simulink model "CHB_3phaseSVPWM_Phaseshift"  (R2015a)
settings: Solver=ode45  StartTime=0.0  StopTime=0.2  MaxStep=0.000001  MinStep=0.0000001  RelTol=1e-3
libraries: powerlib x33, simulink x1
settings Model: Creator=hp  LastModifiedBy=hp

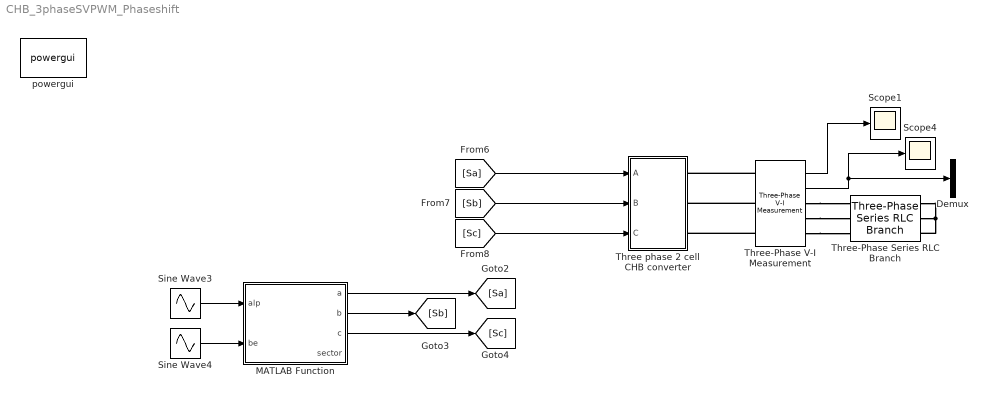
== system CHB_3phaseSVPWM_Phaseshift ==
  Demux : Demux  Outputs=3
  MATLAB Function : MATLAB Function  TreatAsAtomicUnit=on
  Scope1 : Scope
      settings: YMin=-400  YMax=400
  Scope4 : Scope
      settings: YMin=-22.5  YMax=22.5  SaveName=ScopeData5
  Sine Wave3 : Sin  Amplitude=1.0  Frequency=2*pi*50  SampleTime=0
  Sine Wave4 : Sin  Amplitude=1.0  Frequency=2*pi*50  Phase=pi/2  SampleTime=0
  Three phase 2 cell CHB converter : Subsystem
  Three-Phase Series RLC Branch : powerlib/Elements/Three-Phase Series RLC Branch  LConnTagsString=A|B|C  RConnTagsString=A|B|C  BranchType=RLC  Resistance=10  Inductance=10e-3  Capacitance=0  Measurements=None
  Three-Phase V-I Measurement : powerlib/Measurements/Three-Phase V-I Measurement  VoltageMeasurement=phase-to-phase  SetLabelV=off  LabelV=Vabc  Vpu=off  VpuLL=off  CurrentMeasurement=yes  SetLabelI=off  LabelI=Iabc  Ipu=off  Pbase=100e6  Vbase=500e3  OutputType=Complex  PhasorSimulation=off  PSBequivalent=0
  powergui : powerlib/powergui  Priority=1  SimulationMode=Continuous  SolverType=Tustin/Backward Euler (TBE)  SampleTime=50e-6  frequency=60  SPID=off  DisableSnubberDevices=off  DisableRonSwitches=off  DisableVfSwitches=off  SwTol=0  DisplayEquations=off  Interpol=off  methode=off  Ts=100  FunctionMessages=off  echomessages=off  HookPort=off  EnableUseOfTLC=off  x0status=blocks  frequencyindice=0  Pbase=100e6  ErrMax=1e-4  Iterations=50  UnitsV=kV  UnitsW=MW  buscounter=0  RestoreLinks=warning  ResistiveCurrentMeasurement=off  Frange=[0:2:500]  Ylog=off  Xlog=on  ShowGrid=off  save=off  variable=ZData  structure=0  ZoomFFT=off  StartTime=0.0  cycles=1  DisplayStyle=1  fundamental=60  FreqAxis=off  MaxFrequency=1000  frequencyindicesteady=1  RmsSteady=1  display=off
  wires:
  MATLAB Function/1(a) -> [Sa]
  MATLAB Function/2(b) -> [Sb]
  Sine Wave3/1 -> MATLAB Function/1(alp)
  Sine Wave4/1 -> MATLAB Function/2(be)
  MATLAB Function/3(c) -> [Sc]
  Three-Phase V-I Measurement/2 -> Scope4/1, Demux/1
  [Sa] -> Three phase 2 cell CHB converter/1(A)
  [Sb] -> Three phase 2 cell CHB converter/2(B)
  [Sc] -> Three phase 2 cell CHB converter/3(C)
  Three-Phase V-I Measurement/1 -> Scope1/1
  connections:
  Three-Phase Series RLC Branch/RConn1 -- Three-Phase Series RLC Branch/RConn2 -- Three-Phase Series RLC Branch/RConn3
  Three-Phase V-I Measurement/RConn1 -- Three-Phase Series RLC Branch/LConn1
  Three-Phase V-I Measurement/RConn2 -- Three-Phase Series RLC Branch/LConn2
  Three-Phase V-I Measurement/RConn3 -- Three-Phase Series RLC Branch/LConn3
  Three-Phase V-I Measurement/LConn1 -- Three phase 2 cell CHB converter/RConn1
  Three-Phase V-I Measurement/LConn2 -- Three phase 2 cell CHB converter/RConn2
  Three-Phase V-I Measurement/LConn3 -- Three phase 2 cell CHB converter/RConn3

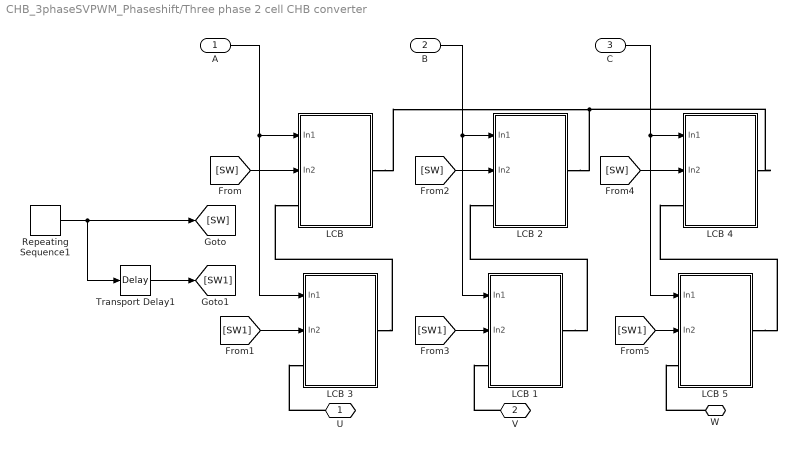
== system CHB_3phaseSVPWM_Phaseshift/Three phase 2 cell CHB converter ==
  A : Inport
  B : Inport  Port=2
  C : Inport  Port=3
  "LCB " : Subsystem
  LCB 1 : Subsystem
  LCB 2 : Subsystem
  LCB 3 : Subsystem
  LCB 4 : Subsystem
  LCB 5 : Subsystem
  Repeating Sequence1 : simulink/Sources/Repeating Sequence  rep_seq_t=[0 0.5 1]/1000  rep_seq_y=[0 1 0]
  Transport Delay1 : TransportDelay  DelayTime=1/4000
  U : PMIOPort  Port=1  Side=Right
  V : PMIOPort  Port=2  Side=Right
  W : PMIOPort  Port=3  Side=Right
  wires:
  [SW1] -> LCB 3/2(In2)
  [SW1] -> LCB 5/2(In2)
  A/1 -> LCB 3/1(In1), "LCB "/1(In1)
  [SW] -> LCB 2/2(In2)
  Repeating Sequence1/1 -> Transport Delay1/1, [SW]
  C/1 -> LCB 4/1(In1), LCB 5/1(In1)
  [SW] -> "LCB "/2(In2)
  [SW1] -> LCB 1/2(In2)
  Transport Delay1/1 -> [SW1]
  B/1 -> LCB 1/1(In1), LCB 2/1(In1)
  [SW] -> LCB 4/2(In2)
  connections:
  "LCB "/RConn1 -- LCB 4/RConn1 -- LCB 2/RConn1
  LCB 3/RConn1 -- "LCB "/LConn1
  LCB 1/RConn1 -- LCB 2/LConn1
  U/RConn1 -- LCB 3/LConn1
  LCB 5/RConn1 -- LCB 4/LConn1
  V/RConn1 -- LCB 1/LConn1
  W/RConn1 -- LCB 5/LConn1

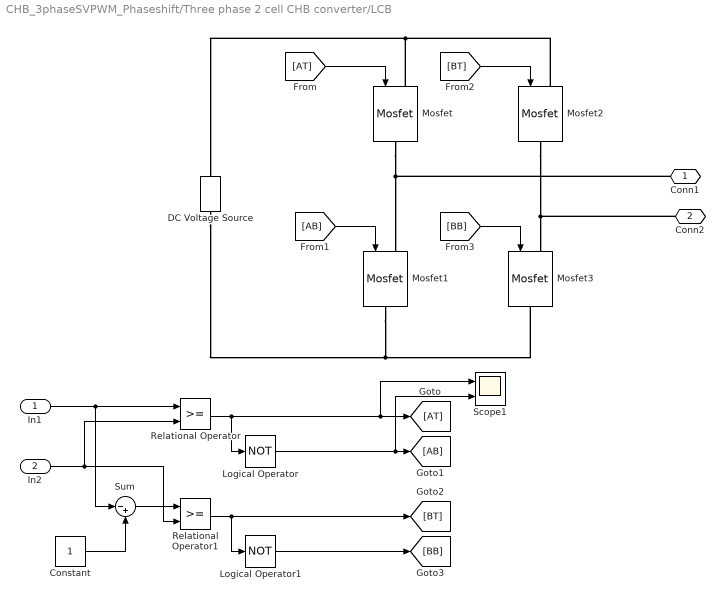
== system CHB_3phaseSVPWM_Phaseshift/Three phase 2 cell CHB converter/LCB  ==
  In1 : Inport
  In2 : Inport  Port=2
  Constant : Constant
  DC Voltage Source : powerlib/Electrical Sources/DC Voltage Source  Amplitude=100  Measurements=None
  Logical Operator : Logic  Operator=NOT  Inputs=1  AllPortsSameDT=off  OutDataTypeStr=boolean
  Logical Operator1 : Logic  Operator=NOT  Inputs=1  AllPortsSameDT=off  OutDataTypeStr=boolean
  Mosfet{,1..3} (4 alike) : powerlib/Power Electronics/Mosfet  Ron=0.1  Lon=0  Rd=0.01  Vfd=0  IC=0  Rs=1e5  Cs=inf  Measurements=off
  Relational Operator : RelationalOperator  OutDataTypeStr=boolean
  Relational Operator1 : RelationalOperator  OutDataTypeStr=boolean
  Scope1 : Scope  NumInputPorts=2
      settings: YMin=-80~-5  YMax=80~5
  Sum : Sum  Inputs=|-+
  Conn1 : PMIOPort  Port=1  Side=Right
  Conn2 : PMIOPort  Port=2  Side=Left
  wires:
  Sum/1 -> Relational Operator1/1
  Relational Operator/1 -> Scope1/1, [AT], Logical Operator/1
  Logical Operator/1 -> Scope1/2, [AB]
  Relational Operator1/1 -> [BT], Logical Operator1/1
  Logical Operator1/1 -> [BB]
  [BB] -> Mosfet3/1
  [AB] -> Mosfet1/1
  [AT] -> Mosfet/1
  [BT] -> Mosfet2/1
  In2/1 -> Relational Operator1/2, Relational Operator/2
  In1/1 -> Sum/1, Relational Operator/1
  Constant/1 -> Sum/2
  connections:
  Mosfet2/RConn1 -- Conn2/RConn1 -- Mosfet3/LConn1
  DC Voltage Source/LConn1 -- Mosfet1/RConn1 -- Mosfet3/RConn1
  Mosfet2/LConn1 -- Mosfet/LConn1 -- DC Voltage Source/RConn1
  Mosfet/RConn1 -- Conn1/RConn1 -- Mosfet1/LConn1

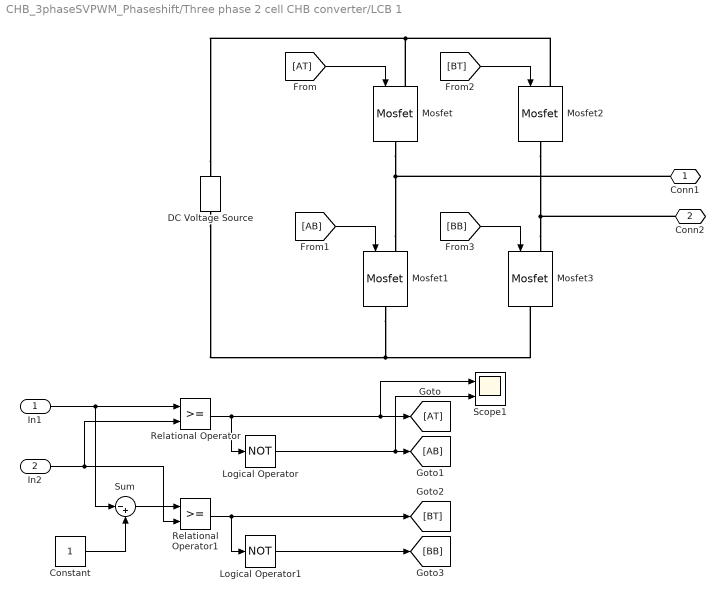
== system CHB_3phaseSVPWM_Phaseshift/Three phase 2 cell CHB converter/LCB 1 ==
  In1 : Inport
  In2 : Inport  Port=2
  Constant : Constant
  DC Voltage Source : powerlib/Electrical Sources/DC Voltage Source  Amplitude=100  Measurements=None
  Logical Operator : Logic  Operator=NOT  Inputs=1  AllPortsSameDT=off  OutDataTypeStr=boolean
  Logical Operator1 : Logic  Operator=NOT  Inputs=1  AllPortsSameDT=off  OutDataTypeStr=boolean
  Mosfet{,1..3} (4 alike) : powerlib/Power Electronics/Mosfet  Ron=0.1  Lon=0  Rd=0.01  Vfd=0  IC=0  Rs=1e5  Cs=inf  Measurements=off
  Relational Operator : RelationalOperator  OutDataTypeStr=boolean
  Relational Operator1 : RelationalOperator  OutDataTypeStr=boolean
  Scope1 : Scope  NumInputPorts=2
      settings: YMin=-80~-5  YMax=80~5
  Sum : Sum  Inputs=|-+
  Conn1 : PMIOPort  Port=1  Side=Right
  Conn2 : PMIOPort  Port=2  Side=Left
  wires:
  Constant/1 -> Sum/2
  In1/1 -> Relational Operator/1, Sum/1
  In2/1 -> Relational Operator/2, Relational Operator1/2
  [BT] -> Mosfet2/1
  [AT] -> Mosfet/1
  [AB] -> Mosfet1/1
  [BB] -> Mosfet3/1
  Logical Operator1/1 -> [BB]
  Relational Operator1/1 -> Logical Operator1/1, [BT]
  Logical Operator/1 -> [AB], Scope1/2
  Relational Operator/1 -> Logical Operator/1, [AT], Scope1/1
  Sum/1 -> Relational Operator1/1
  connections:
  Mosfet1/LConn1 -- Conn1/RConn1 -- Mosfet/RConn1
  DC Voltage Source/RConn1 -- Mosfet/LConn1 -- Mosfet2/LConn1
  Mosfet3/RConn1 -- Mosfet1/RConn1 -- DC Voltage Source/LConn1
  Mosfet3/LConn1 -- Conn2/RConn1 -- Mosfet2/RConn1

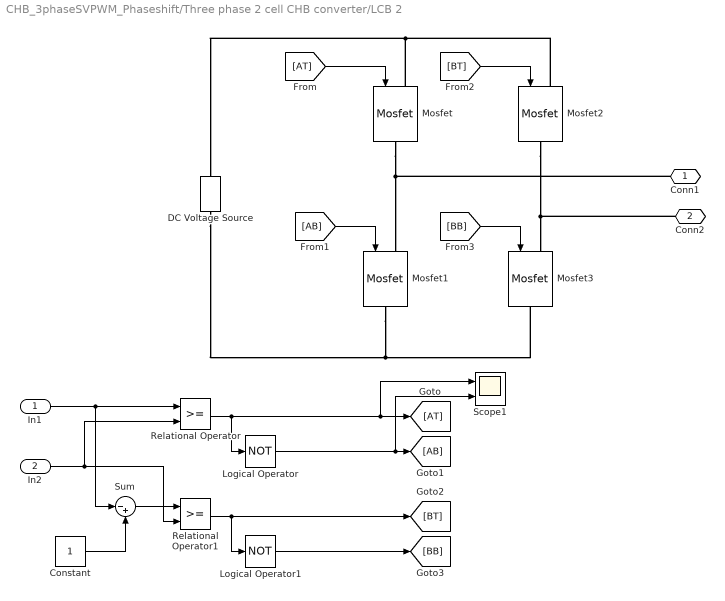
== system CHB_3phaseSVPWM_Phaseshift/Three phase 2 cell CHB converter/LCB 2 ==
  In1 : Inport
  In2 : Inport  Port=2
  Constant : Constant
  DC Voltage Source : powerlib/Electrical Sources/DC Voltage Source  Amplitude=100  Measurements=None
  Logical Operator : Logic  Operator=NOT  Inputs=1  AllPortsSameDT=off  OutDataTypeStr=boolean
  Logical Operator1 : Logic  Operator=NOT  Inputs=1  AllPortsSameDT=off  OutDataTypeStr=boolean
  Mosfet{,1..3} (4 alike) : powerlib/Power Electronics/Mosfet  Ron=0.1  Lon=0  Rd=0.01  Vfd=0  IC=0  Rs=1e5  Cs=inf  Measurements=off
  Relational Operator : RelationalOperator  OutDataTypeStr=boolean
  Relational Operator1 : RelationalOperator  OutDataTypeStr=boolean
  Scope1 : Scope  NumInputPorts=2
      settings: YMin=-80~-5  YMax=80~5
  Sum : Sum  Inputs=|-+
  Conn1 : PMIOPort  Port=1  Side=Right
  Conn2 : PMIOPort  Port=2  Side=Left
  wires:
  Sum/1 -> Relational Operator1/1
  Relational Operator/1 -> Scope1/1, [AT], Logical Operator/1
  Logical Operator/1 -> Scope1/2, [AB]
  Relational Operator1/1 -> [BT], Logical Operator1/1
  Logical Operator1/1 -> [BB]
  [BB] -> Mosfet3/1
  [AB] -> Mosfet1/1
  [AT] -> Mosfet/1
  [BT] -> Mosfet2/1
  In2/1 -> Relational Operator1/2, Relational Operator/2
  In1/1 -> Sum/1, Relational Operator/1
  Constant/1 -> Sum/2
  connections:
  Mosfet2/RConn1 -- Conn2/RConn1 -- Mosfet3/LConn1
  DC Voltage Source/LConn1 -- Mosfet1/RConn1 -- Mosfet3/RConn1
  Mosfet2/LConn1 -- Mosfet/LConn1 -- DC Voltage Source/RConn1
  Mosfet/RConn1 -- Conn1/RConn1 -- Mosfet1/LConn1

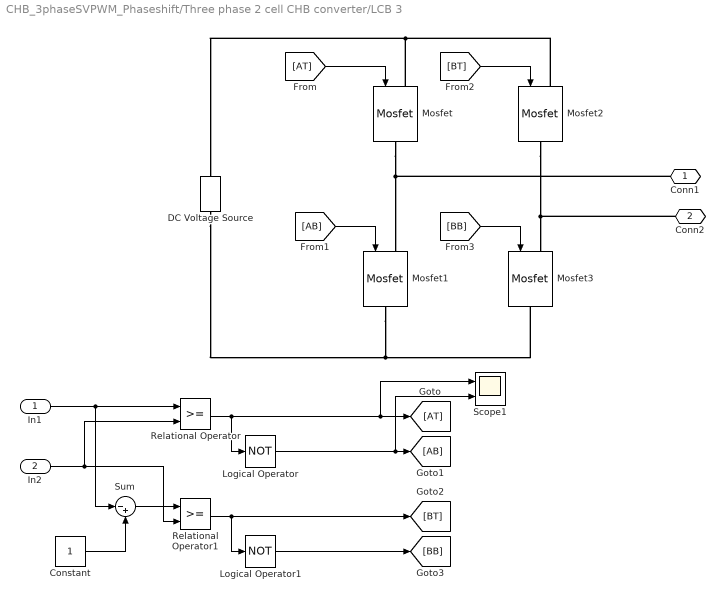
== system CHB_3phaseSVPWM_Phaseshift/Three phase 2 cell CHB converter/LCB 3 ==
  In1 : Inport
  In2 : Inport  Port=2
  Constant : Constant
  DC Voltage Source : powerlib/Electrical Sources/DC Voltage Source  Amplitude=100  Measurements=None
  Logical Operator : Logic  Operator=NOT  Inputs=1  AllPortsSameDT=off  OutDataTypeStr=boolean
  Logical Operator1 : Logic  Operator=NOT  Inputs=1  AllPortsSameDT=off  OutDataTypeStr=boolean
  Mosfet{,1..3} (4 alike) : powerlib/Power Electronics/Mosfet  Ron=0.1  Lon=0  Rd=0.01  Vfd=0  IC=0  Rs=1e5  Cs=inf  Measurements=off
  Relational Operator : RelationalOperator  OutDataTypeStr=boolean
  Relational Operator1 : RelationalOperator  OutDataTypeStr=boolean
  Scope1 : Scope  NumInputPorts=2
      settings: YMin=-80~-5  YMax=80~5
  Sum : Sum  Inputs=|-+
  Conn1 : PMIOPort  Port=1  Side=Right
  Conn2 : PMIOPort  Port=2  Side=Left
  wires:
  Sum/1 -> Relational Operator1/1
  Relational Operator/1 -> Scope1/1, [AT], Logical Operator/1
  Logical Operator/1 -> Scope1/2, [AB]
  Relational Operator1/1 -> [BT], Logical Operator1/1
  Logical Operator1/1 -> [BB]
  [BB] -> Mosfet3/1
  [AB] -> Mosfet1/1
  [AT] -> Mosfet/1
  [BT] -> Mosfet2/1
  In2/1 -> Relational Operator1/2, Relational Operator/2
  In1/1 -> Sum/1, Relational Operator/1
  Constant/1 -> Sum/2
  connections:
  Mosfet2/RConn1 -- Conn2/RConn1 -- Mosfet3/LConn1
  DC Voltage Source/LConn1 -- Mosfet1/RConn1 -- Mosfet3/RConn1
  Mosfet2/LConn1 -- Mosfet/LConn1 -- DC Voltage Source/RConn1
  Mosfet/RConn1 -- Conn1/RConn1 -- Mosfet1/LConn1

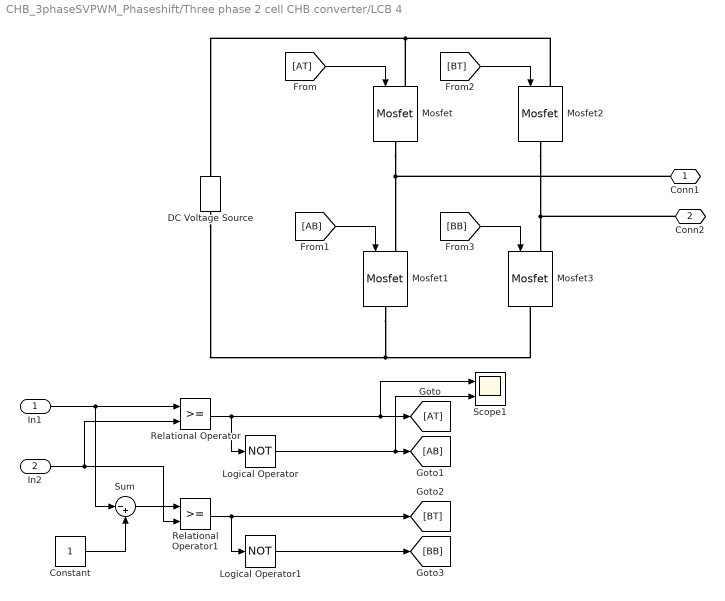
== system CHB_3phaseSVPWM_Phaseshift/Three phase 2 cell CHB converter/LCB 4 ==
  In1 : Inport
  In2 : Inport  Port=2
  Constant : Constant
  DC Voltage Source : powerlib/Electrical Sources/DC Voltage Source  Amplitude=100  Measurements=None
  Logical Operator : Logic  Operator=NOT  Inputs=1  AllPortsSameDT=off  OutDataTypeStr=boolean
  Logical Operator1 : Logic  Operator=NOT  Inputs=1  AllPortsSameDT=off  OutDataTypeStr=boolean
  Mosfet{,1..3} (4 alike) : powerlib/Power Electronics/Mosfet  Ron=0.1  Lon=0  Rd=0.01  Vfd=0  IC=0  Rs=1e5  Cs=inf  Measurements=off
  Relational Operator : RelationalOperator  OutDataTypeStr=boolean
  Relational Operator1 : RelationalOperator  OutDataTypeStr=boolean
  Scope1 : Scope  NumInputPorts=2
      settings: YMin=-80~-5  YMax=80~5
  Sum : Sum  Inputs=|-+
  Conn1 : PMIOPort  Port=1  Side=Right
  Conn2 : PMIOPort  Port=2  Side=Left
  wires:
  Sum/1 -> Relational Operator1/1
  Relational Operator/1 -> Scope1/1, [AT], Logical Operator/1
  Logical Operator/1 -> Scope1/2, [AB]
  Relational Operator1/1 -> [BT], Logical Operator1/1
  Logical Operator1/1 -> [BB]
  [BB] -> Mosfet3/1
  [AB] -> Mosfet1/1
  [AT] -> Mosfet/1
  [BT] -> Mosfet2/1
  In2/1 -> Relational Operator1/2, Relational Operator/2
  In1/1 -> Sum/1, Relational Operator/1
  Constant/1 -> Sum/2
  connections:
  Mosfet2/RConn1 -- Conn2/RConn1 -- Mosfet3/LConn1
  DC Voltage Source/LConn1 -- Mosfet1/RConn1 -- Mosfet3/RConn1
  Mosfet2/LConn1 -- Mosfet/LConn1 -- DC Voltage Source/RConn1
  Mosfet/RConn1 -- Conn1/RConn1 -- Mosfet1/LConn1

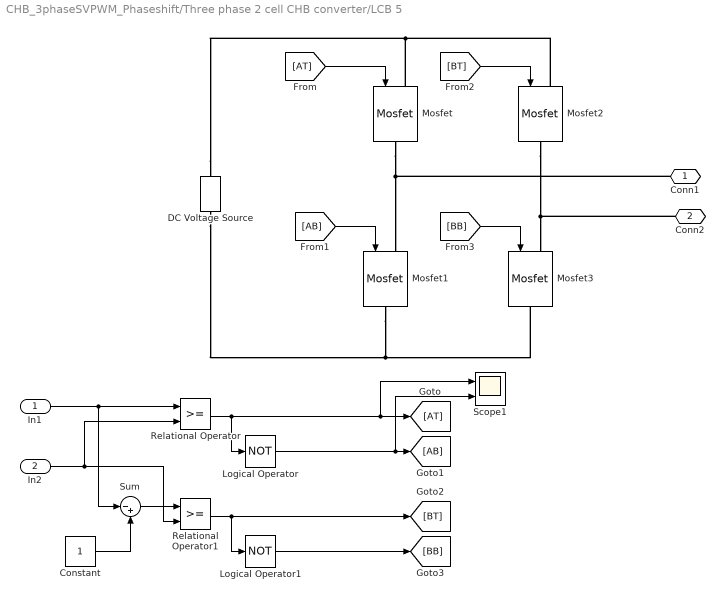
== system CHB_3phaseSVPWM_Phaseshift/Three phase 2 cell CHB converter/LCB 5 ==
  In1 : Inport
  In2 : Inport  Port=2
  Constant : Constant
  DC Voltage Source : powerlib/Electrical Sources/DC Voltage Source  Amplitude=100  Measurements=None
  Logical Operator : Logic  Operator=NOT  Inputs=1  AllPortsSameDT=off  OutDataTypeStr=boolean
  Logical Operator1 : Logic  Operator=NOT  Inputs=1  AllPortsSameDT=off  OutDataTypeStr=boolean
  Mosfet{,1..3} (4 alike) : powerlib/Power Electronics/Mosfet  Ron=0.1  Lon=0  Rd=0.01  Vfd=0  IC=0  Rs=1e5  Cs=inf  Measurements=off
  Relational Operator : RelationalOperator  OutDataTypeStr=boolean
  Relational Operator1 : RelationalOperator  OutDataTypeStr=boolean
  Scope1 : Scope  NumInputPorts=2
      settings: YMin=-80~-5  YMax=80~5
  Sum : Sum  Inputs=|-+
  Conn1 : PMIOPort  Port=1  Side=Right
  Conn2 : PMIOPort  Port=2  Side=Left
  wires:
  Sum/1 -> Relational Operator1/1
  Relational Operator/1 -> Scope1/1, [AT], Logical Operator/1
  Logical Operator/1 -> Scope1/2, [AB]
  Relational Operator1/1 -> [BT], Logical Operator1/1
  Logical Operator1/1 -> [BB]
  [BB] -> Mosfet3/1
  [AB] -> Mosfet1/1
  [AT] -> Mosfet/1
  [BT] -> Mosfet2/1
  In2/1 -> Relational Operator1/2, Relational Operator/2
  In1/1 -> Sum/1, Relational Operator/1
  Constant/1 -> Sum/2
  connections:
  Mosfet2/RConn1 -- Conn2/RConn1 -- Mosfet3/LConn1
  Mosfet3/RConn1 -- DC Voltage Source/LConn1 -- Mosfet1/RConn1
  DC Voltage Source/RConn1 -- Mosfet2/LConn1 -- Mosfet/LConn1
  Mosfet/RConn1 -- Mosfet1/LConn1 -- Conn1/RConn1

== matlab function CHB_3phaseSVPWM_Phaseshift/MATLAB Function ==
  data: alp input; a output; be input; b output; c output; sector output
function [a,b,c,sector] = fcn(alp,be)
%#codegen
	sec_a=0,sec_b=0,sec_c=0;
	t_o = 0,ta = 0,tb = 0,tc = 0,tsec = 0;

    sec_a = be;										%Beta;
	sec_b = ((-be/2)+(alp*0.866));			%(-0.5*Beta+(0.866*alpha));
	sec_c = ((-be/2)-(alp*0.866));			%(-0.5*Beta-(0.866*alpha));
    
    if(sec_a>=0)
       if(sec_b>=0)
       												%	sector 1
    		t_o = (1 - (sec_a+sec_b))/2;							%	t_1 = sec_b, t_2 =sec_a
    		ta = sec_a+sec_b+(t_o);
    		tb  = sec_a+(t_o);
    		tc  = (t_o);
            tsec = 1;
       else
            if(sec_c>=0)												%	sector 3
        		t_o = (1 - (sec_a+sec_c))/2;						%	t_1 = sec_a, t_2 =sec_c
        		ta = (t_o);
        		tb = sec_a+sec_c+(t_o);
        		tc = sec_c+(t_o);
                tsec = 3;
            else												%	sector 2
        		t_o = (1 + (sec_c+sec_b))/2;					%	t_1 = -sec_c, t_2 =-sec_b
        		ta = -sec_c+(t_o);
        		tb = -(sec_c+sec_b)+(t_o);
        		tc = (t_o);
                tsec = 2;
            end
       end
    else
       if(sec_b>=0)
           if(sec_c>=0)                                                  %	sector 5
        		t_o = (1 - (sec_c+sec_b))/2; 				%	t_1 = sec_c, t_2 =sec_b
        		ta = sec_b+(t_o);
        		tb = (t_o);
        		tc = sec_c+sec_b+(t_o);
                tsec = 5;
           else                                                  %	sector 6
        		t_o = (1 + (sec_a+sec_c))/2; 				%	t_1 = -sec_a, t_2 =-sec_c
        		ta = -(sec_a+sec_c)+(t_o);
        		tb = (t_o);
        		tc = -sec_a+(t_o);
                tsec = 6;
           end
       else
            if(sec_c>=0)                                      %	sector 4
        		t_o = (1 + (sec_a+sec_b))/2;			%	t_1 = -sec_b, t_2 =-sec_a
        		ta = (t_o);
        		tb = -sec_b+(t_o);
        		tc = -(sec_a+sec_b)+(t_o);
                tsec = 4;
            end
       end
    end
a = ta;
b = tb;
c = tc;
sector = tsec;
